simulink model "functionSPID"  (R2020b)
settings: Solver=ode4  StartTime=0.0  StopTime=100  RelTol=1e-3
settings Model: Creator=Robert  LastModifiedBy=Robert

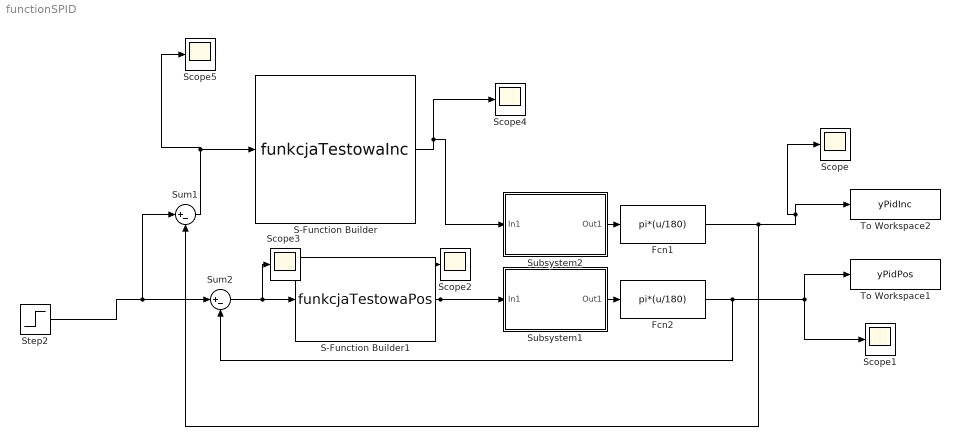
== system functionSPID ==
  Fcn1 : Fcn  Expr=pi*(u/180)
  Fcn2 : Fcn  Expr=pi*(u/180)
  S-Function Builder : S-Function  FunctionName=funkcjaTestowaInc  SFunctionModules=funkcjaTestowaInc_wrapper  SFunctionDeploymentMode=off  EnableBusSupport=off  mask(S-Function Builder){}
      mask help: Simulink:masks:SFunctionBuilder_MD
      mask init:
      | val = [[.9  0.75 0.75 1 1 .9 .9 1]',[1 1 0.75 0.75 .9 .9 1 .9]'];try , sys = get_param(gcb,'SfunBuilderFcnName');if isempty(sys), sys = get_param(gcb,'FunctionName'); end,catch, sys = get_param(gcb,'FunctionName'); end
      settings: CopyFcn=set_param(gcbh,'LinkStatus','none')  OpenFcn=sfunctionwizard(gcbh)
      mask Display:
      | plot(val(:,1),val(:,2))
      | disp(sys)
      | port_label('input',1,'eInc')
      | port_label('output',1,'yInc')
  S-Function Builder1 : S-Function  FunctionName=funkcjaTestowaPos  SFunctionModules=funkcjaTestowaPos_wrapper  SFunctionDeploymentMode=off  EnableBusSupport=off  mask(S-Function Builder){}
      mask help: Simulink:masks:SFunctionBuilder_MD
      mask init: same as functionSPID/S-Function Builder
      settings: CopyFcn=set_param(gcbh,'LinkStatus','none')  OpenFcn=sfunctionwizard(gcbh)
      mask Display:
      | plot(val(:,1),val(:,2))
      | disp(sys)
      | port_label('input',1,'ePos')
      | port_label('output',1,'yPos')
  Scope{,1..5} (6 alike) : Scope
  Step2 : Step  Time=0  After=u  SampleTime=0
  Subsystem1 : Subsystem
  Subsystem2 : Subsystem
  Sum1 : Sum  Inputs=|+-
  Sum2 : Sum  Inputs=|+-
  To Workspace1 : ToWorkspace  VariableName=yPidPos  SampleTime=-1
      settings: Save2DSignal=2-D array (concatenate along first dimension)
  To Workspace2 : ToWorkspace  VariableName=yPidInc  SampleTime=-1
      settings: Save2DSignal=2-D array (concatenate along first dimension)
  wires:
  Step2/1 -> Sum1/1, Sum2/1
  Fcn2/1 -> Sum2/2, Scope1/1, To Workspace1/1
  Subsystem1/1(Out1) -> Fcn2/1
  Fcn1/1 -> Scope/1, To Workspace2/1, Sum1/2
  Subsystem2/1(Out1) -> Fcn1/1
  Sum1/1 -> Scope5/1, S-Function Builder/1
  S-Function Builder/1 -> Scope4/1, Subsystem2/1(In1)
  Sum2/1 -> Scope3/1, S-Function Builder1/1
  S-Function Builder1/1 -> Subsystem1/1(In1), Scope2/1

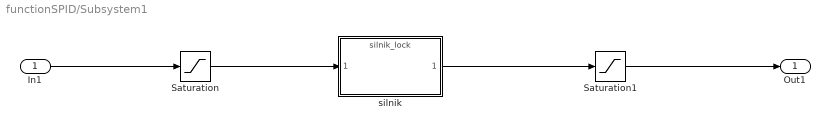
== system functionSPID/Subsystem1 ==
  In1 : Inport
  Saturation : Saturate  UpperLimit=2  LowerLimit=-2
  Saturation1 : Saturate  UpperLimit=180  LowerLimit=-180
  silnik : ModelReference  ModelNameDialog=silnik_lock.slxp  ModelReferenceVersion=1.38  CopyOfModelProtected=on
  Out1 : Outport
  wires:
  Saturation/1 -> silnik/1
  In1/1 -> Saturation/1
  silnik/1 -> Saturation1/1
  Saturation1/1 -> Out1/1

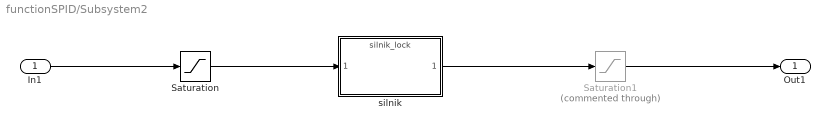
== system functionSPID/Subsystem2 ==
  In1 : Inport
  Saturation : Saturate  UpperLimit=2  LowerLimit=-2
  Saturation1 : Saturate  Commented=through  UpperLimit=180  LowerLimit=-180
  silnik : ModelReference  ModelNameDialog=silnik_lock.slxp  ModelReferenceVersion=1.38  CopyOfModelProtected=on
  Out1 : Outport
  wires:
  Saturation/1 -> silnik/1
  In1/1 -> Saturation/1
  silnik/1 -> Saturation1/1
  Saturation1/1 -> Out1/1
